simulink model "LFSRexterior"  (R2019a)
settings: Solver=VariableStepAuto  StartTime=0.0  StopTime=10.0  RelTol=1e-3
settings Model: Creator=Maftei Silviu  LastModifiedBy=Maftei Silviu

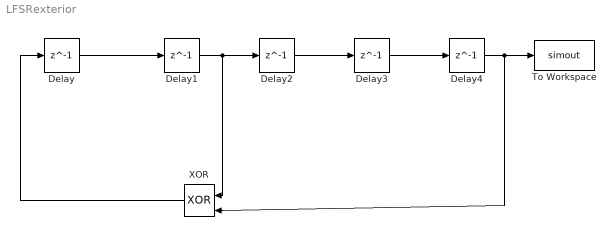
== system LFSRexterior ==
  Delay : Delay  DelayLength=1  InitialCondition=1
  Delay{1..4} (4 alike) : Delay  DelayLength=1  InitialCondition=0
  To Workspace : ToWorkspace  VariableName=simout  SampleTime=-1
      settings: Save2DSignal=2-D array (concatenate along first dimension)
  XOR : Logic  Operator=XOR  IconShape=distinctive  AllPortsSameDT=off  OutDataTypeStr=boolean
  wires:
  XOR/1 -> Delay/1
  Delay/1 -> Delay1/1
  Delay1/1 -> XOR/1, Delay2/1
  Delay2/1 -> Delay3/1
  Delay3/1 -> Delay4/1
  Delay4/1 -> XOR/2, To Workspace/1
